simulink model "ElasticPendulum"  (R2017b)
settings: Solver=ode45  StartTime=0.0  StopTime=10  MaxStep=.01  RelTol=1e-11  AbsTol=1e-11  EnableMultiTasking=on
values from neighbouring files (symbols this model uses):
  g = 9.81    [BigSweep2.m]    (also in ElasticPendulum2.m; NoiseAmbient.m; Original_running_params.m; TheGoodBand.m)
  k = 12000    [ElasticPendulum2.m]    (also in Original_running_params.m = 20000)
  l0 = 1    [BigSweep2.m]    (also in ElasticPendulum2.m; NoiseAmbient.m; Original_running_params.m; TheGoodBand.m)
  m = 80    [BigSweep2.m]    (also in ElasticPendulum2.m; NoiseAmbient.m; Original_running_params.m; TheGoodBand.m)
  Vx0 = real((2/m*(Esys-m*g*(y0-yG)))^.5)    [BigSweep2.m]    (also in ElasticPendulum2.m = 2.11026064741; NoiseAmbient.m = 2.11; TheGoodBand.m = 2.11)
  Vy0 = 0    [BigSweep2.m]    (also in ElasticPendulum2.m; NoiseAmbient.m; TheGoodBand.m)
  x0 = []    [AnimSMR.m]    (also in BigSweep2.m = 3; ElasticPendulum2.m = -0.2; NoiseAmbient.m = 3; Original_running_params.m = 0)
  y0 = Y0minEver+(yMaxRel-Y0minEver)*NyCycle/Ny    [BigSweep2.m]    (also in ElasticPendulum2.m = 0.98; NoiseAmbient.m = 0.98; Original_running_params.m = 1; TheGoodBand.m = 0.98)
  yG = 0    [BigSweep2.m]    (also in ElasticPendulum2.m; NoiseAmbient.m; Original_running_params.m; TheGoodBand.m)
libraries: simulink x8
settings Model: Creator=hgeyer  LastModifiedBy=jfr
settings DataIOCC: LimitDataPoints=on  SaveFormat=Array
settings OptimizationCC: ExpressionDepthLimit=2147483647  LifeSpan=inf
settings DebuggingCC: UnderspecifiedInitializationDetection=Classic  MergeDetectMultiDrivingBlocksExec=none  SolverPrmCheckMsg=warning  StateNameClashWarn=warning  SFUnexpectedBacktrackingDiag=warning  SFNoUnconditionalDefaultTransitionDiag=warning  SFExecutionAtInitializationDiag=none
settings HardwareCC: ProdBitPerPointer=32  ProdBitPerSizeT=32  ProdBitPerPtrDiffT=32  ProdLargestAtomicFloat=None  ProdIntDivRoundTo=Undefined  ProdEndianess=Unspecified  ProdWordSize=32  ProdHWDeviceType=32-bit Generic
settings ModelReferenceCC: PropagateSignalLabelsOutOfModel=off
settings CodeAppCC: StateflowObjectComments=on
settings GRTTargetCC: TargetLangStandard=C89/C90 (ANSI)  GeneratePreprocessorConditionals=Disable all
settings ConfigComp: CovMetricSettings=dw  CovHtmlReporting=on  CovSaveCumulativeToWorkspaceVar=on  CovSaveSingleToWorkspaceVar=on  CovExternalEMLEnable=off

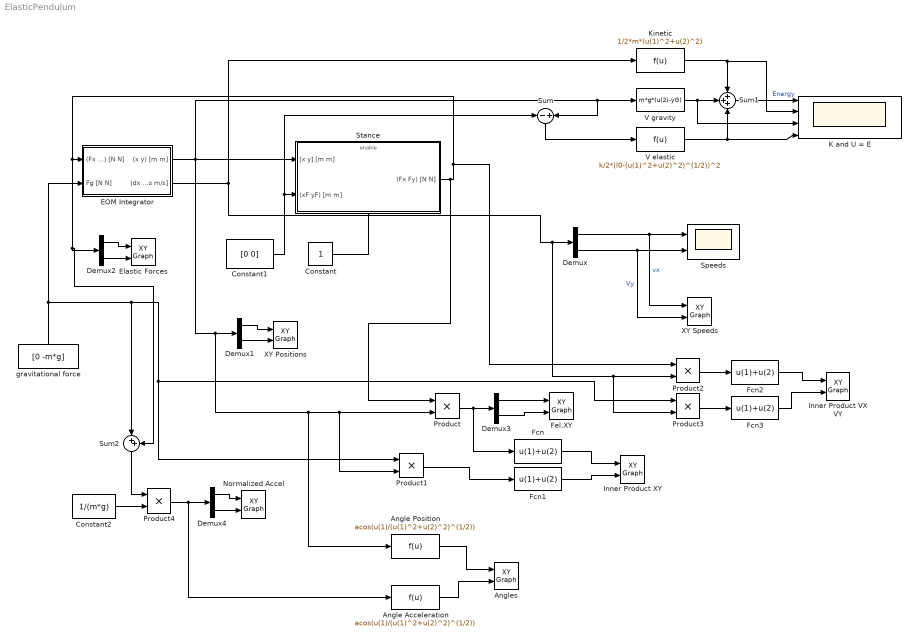
== system ElasticPendulum ==
  Angle Acceleration : Fcn  Expr=acos(u(1)/(u(1)^2+u(2)^2)^(1/2))
  Angle Position : Fcn  Expr=acos(u(1)/(u(1)^2+u(2)^2)^(1/2))
  Angles : simulink/Sinks/XY Graph  xmin=-2*pi  xmax=2*pi  ymin=-2*pi  ymax=2*pi  st=-1
  Constant : Constant
  Constant1 : Constant  Value=[0 0]
  Constant2 : Constant  Value=1/(m*g)
  Demux{,1..4} (5 alike) : Demux  Outputs=2
  EOM Integrator : Subsystem
  Elastic Forces : simulink/Sinks/XY Graph  xmin=-8000  xmax=8000  ymin=-8000  ymax=8000  st=-1
  Fcn{,1..3} (4 alike) : Fcn  Expr=u(1)+u(2)
  Fel.XY : simulink/Sinks/XY Graph  xmin=-12500  xmax=12500  ymin=-12500  ymax=12500  st=-1
  Inner Product VX VY : simulink/Sinks/XY Graph  xmin=-12500  xmax=12500  ymin=-12500  ymax=12500  st=-1
  Inner Product XY : simulink/Sinks/XY Graph  xmin=-5500  xmax=5500  ymin=-5500  ymax=5500  st=-1
  K and U = E : Scope  NumInputPorts=4
  Kinetic : Fcn  Expr=1/2*m*(u(1)^2+u(2)^2)
  Normalized Accel : simulink/Sinks/XY Graph  xmin=-8  xmax=8  ymin=-8  ymax=8  st=-1
  Product{,1..4} (5 alike) : Product
  Speeds : Scope  NumInputPorts=2
  Stance : Subsystem
  Sum : Sum  Inputs=-+
  Sum1 : Sum  Inputs=3
  Sum2 : Sum  Inputs=|++
  V elastic : Fcn  Expr=k/2*(l0-(u(1)^2+u(2)^2)^(1/2))^2
  V gravity : Fcn  Expr=m*g*(u(2)-yG)
  XY Positions : simulink/Sinks/XY Graph  xmin=-2  xmax=2  ymin=-2  ymax=2  st=-1
  XY Speeds : simulink/Sinks/XY Graph  xmin=-10  xmax=10  ymin=-10  ymax=10  st=-1
  gravitational force : Constant  Value=[0 -m*g]
  wires:
  Sum1/1 -> K and U = E/1  "Energy"
  V elastic/1 -> Sum1/3, K and U = E/4
  EOM Integrator/2((dx dy) [m/s m/s]) -> Product3/2, Product2/2, Demux/1, Kinetic/1
  Demux/2 -> XY Speeds/2, Speeds/2  "Vy"
  V gravity/1 -> K and U = E/3, Sum1/2
  Sum/1 -> V elastic/1
  Kinetic/1 -> K and U = E/2, Sum1/1
  EOM Integrator/1((x y) [m m]) -> Angle Position/1, Product1/2, Product/2, Demux1/1, Sum/2, V gravity/1, Stance/1("[x y] [m m]")
  Demux/1 -> XY Speeds/1, Speeds/1  "vx"
  Constant/1 -> Stance/Enable
  Demux2/1 -> Elastic Forces/1
  Demux2/2 -> Elastic Forces/2
  Constant1/1 -> Sum/1, Stance/2((xF yF) [m m])
  Demux1/2 -> XY Positions/2
  Demux1/1 -> XY Positions/1
  gravitational force/1 -> Product3/1, Product1/1, Sum2/1, EOM Integrator/2(Fg [N N])
  Product/1 -> Fcn/1, Demux3/1
  Demux3/1 -> Fel.XY/1
  Demux3/2 -> Fel.XY/2
  Fcn/1 -> Inner Product XY/1
  Product1/1 -> Fcn1/1
  Fcn1/1 -> Inner Product XY/2
  Product2/1 -> Fcn2/1
  Product3/1 -> Fcn3/1
  Fcn2/1 -> Inner Product VX VY/1
  Fcn3/1 -> Inner Product VX VY/2
  Demux4/2 -> Normalized Accel/2
  Demux4/1 -> Normalized Accel/1
  Stance/1((Fx Fy) [N N]) -> Product/1, Product2/1, Sum2/2, Demux2/1, EOM Integrator/1((Fx Fy) [N N])
  Sum2/1 -> Product4/1
  Product4/1 -> Angle Acceleration/1, Demux4/1
  Constant2/1 -> Product4/2
  Angle Position/1 -> Angles/1
  Angle Acceleration/1 -> Angles/2

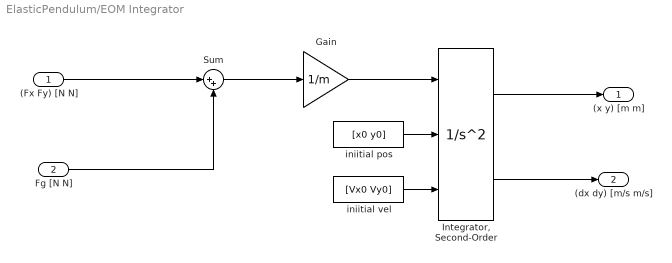
== system ElasticPendulum/EOM Integrator ==
  (Fx Fy) [N N] : Inport
  Fg [N N] : Inport  Port=2
  Gain : Gain  Gain=1/m
  "Integrator, Second-Order" : SecondOrderIntegrator  ICSourceX=external  ICSourceDXDT=external
  Sum : Sum  Inputs=|++
  iniitial pos : Constant  Value=[x0 y0]
  iniitial vel : Constant  Value=[Vx0 Vy0]
  (x y) [m m] : Outport
  (dx dy) [m/s m/s] : Outport  Port=2
  wires:
  Gain/1 -> "Integrator, Second-Order"/1
  "Integrator, Second-Order"/1 -> (x y) [m m]/1
  iniitial vel/1 -> "Integrator, Second-Order"/3
  (Fx Fy) [N N]/1 -> Sum/1
  iniitial pos/1 -> "Integrator, Second-Order"/2
  Sum/1 -> Gain/1
  "Integrator, Second-Order"/2 -> (dx dy) [m/s m/s]/1
  Fg [N N]/1 -> Sum/2

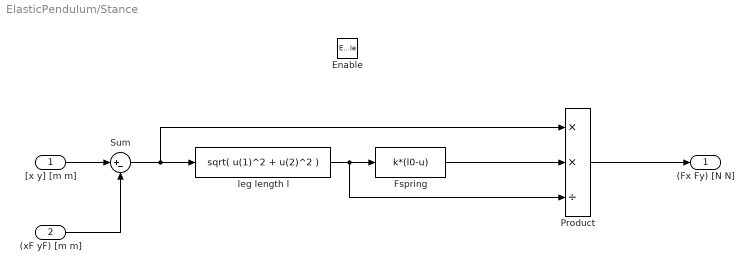
== system ElasticPendulum/Stance ==
  "[x y] [m m]" : Inport
  (xF yF) [m m] : Inport  Port=2
  Enable : EnablePort  StatesWhenEnabling=reset
  Fspring : Fcn  Expr=k*(l0-u)
  Product : Product  Inputs=**/  RndMeth=Zero
  Sum : Sum  Inputs=|+-
  leg length l : Fcn  Expr=sqrt( u(1)^2 + u(2)^2 )
  (Fx Fy) [N N] : Outport  OutputWhenDisabled=reset  InitialOutput=[0 0]
  wires:
  Fspring/1 -> Product/2
  Sum/1 -> Product/1, leg length l/1
  "[x y] [m m]"/1 -> Sum/1
  (xF yF) [m m]/1 -> Sum/2
  Product/1 -> (Fx Fy) [N N]/1
  leg length l/1 -> Fspring/1, Product/3
